simulink model "sdruFMReceiverSimulinkExample"  (R2019a)
settings: Solver=FixedStepDiscrete  StartTime=0.0  StopTime=inf  RelTol=1e-3
PreLoadFcn:
  | platform = sdruExampleFindRadio;
  | stereoFMRxParams = getParamsSdruFMExamples(platform);
  | clear platform
PostLoadFcn:
  | sdruExampleSetAvailableRadio();
InitFcn:
  | platform = get_param([gcs '/SDRu Receiver'], 'Platform');
  | stereoFMRxParams = getParamsSdruFMExamples(platform);
  | clear platform
libraries: simulink x1, dspsnks4 x1, commanabbnd3 x1, sdrublksprivate x1, commsdrhw_v2 x1
Description:
  | This model uses Universal Software Radio Peripheral (USRP) hardware with Simulink(R) to perform FM demodulation and stereo decoding.
settings Model: Creator=The MathWorks, Inc.  LastModifiedBy=ASUS
settings DataIOCC: SaveFormat=Structure  SaveOutput=off  SignalLogging=off  DSMLogging=off  SaveTime=off  ReturnWorkspaceOutputs=off
settings OptimizationCC: ExpressionDepthLimit=2147483647  EfficientMapNaN2IntZero=off  LifeSpan=inf  SimCompilerOptimization=on
settings DebuggingCC: UnderspecifiedInitializationDetection=Classic  MergeDetectMultiDrivingBlocksExec=none  SolverPrmCheckMsg=warning  InheritedTsInSrcMsg=none  MultiTaskCondExecSysMsg=none  ParameterPrecisionLossMsg=none  FcnCallInpInsideContextMsg=warning  AllowSymbolicDim=off  StateNameClashWarn=warning  SFUnexpectedBacktrackingDiag=warning  SFNoUnconditionalDefaultTransitionDiag=warning  SFExecutionAtInitializationDiag=none  ArithmeticOperatorsInVariantConditions=warning
settings HardwareCC: ProdBitPerPointer=32  ProdBitPerSizeT=32  ProdBitPerPtrDiffT=32  ProdLargestAtomicFloat=None  ProdIntDivRoundTo=Undefined  ProdEndianess=Unspecified  ProdWordSize=32  ProdHWDeviceType=32-bit Generic  TargetBitPerPointer=64  TargetBitPerSizeT=64  TargetBitPerPtrDiffT=64  TargetLongLongMode=on  TargetIntDivRoundTo=Zero  TargetEndianess=LittleEndian  TargetWordSize=64  TargetHWDeviceType=Generic->MATLAB Host Computer  ProdEqTarget=off
settings ModelReferenceCC: PropagateSignalLabelsOutOfModel=off
settings SFSimCC: SimIntegrity=off  SimUseLocalCustomCode=off
settings RTWCC: RTWUseLocalCustomCode=off
settings RTWCC: CustomSourceCode=|
  | #include <stdio.h>
  | #include <stdlib.h>
settings CodeAppCC: MaxIdLength=128  StateflowObjectComments=on
settings GRTTargetCC: TargetLangStandard=C89/C90 (ANSI)  GeneratePreprocessorConditionals=Disable all  CombineOutputUpdateFcns=off  GRTInterface=on
settings ConfigComp: CovMetricSettings=dw  CovHtmlReporting=on  CovSaveCumulativeToWorkspaceVar=on  CovSaveSingleToWorkspaceVar=on  CovExternalEMLEnable=off  CovSFcnEnable=off

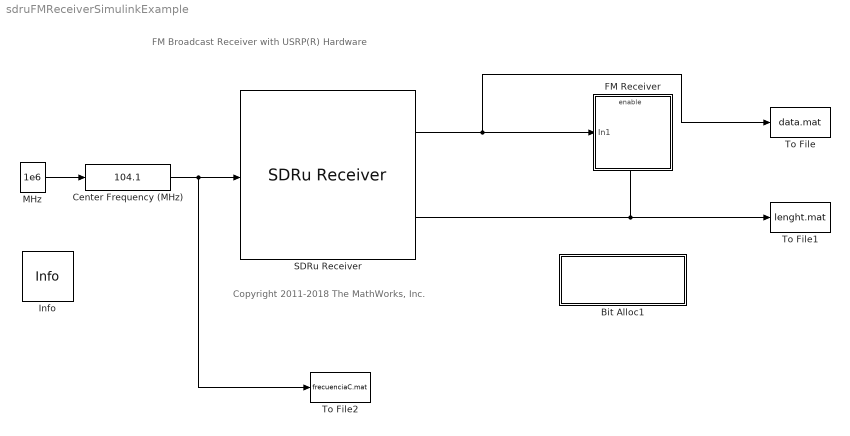
== system sdruFMReceiverSimulinkExample ==
  note: Copyright 2011-2018 The MathWorks, Inc.
  note: FM Broadcast Receiver with USRP(R) Hardware
  Bit Alloc1 : Subsystem
      settings: OpenFcn=sdruFMReceiverMidiSimulinkExample
      mask Display: disp('Alternative version\nwith midi controller\nfor station selection')
  Center Frequency (MHz) : simulink/Math Operations/Slider Gain  gain=104.1  low=87.5  high=108
  FM Receiver : Subsystem  TreatAsAtomicUnit=on
      mask Display:
      | plot(0,0,100,100,[5+4.5*[0:.15:10] 50 50 50 50+4.5*[0:10]],[85+10*[sin([0:.15:10]*pi*2+cumsum(sin([0:.15:10]*pi/5))/2)] 85 99 75   10*sin([0:10]*pi/5)+85])
      | disp('\nFM\nBroadcast\nDemodulator')
  Info : sdrublksprivate/Info  SystemSampleTime=-1
      settings: SourceProductName=Communications Toolbox Support Package for USRP Radio  SourceProductBaseCode=USRP
  MHz : Constant  Value=1e6  VectorParams1D=off  SampleTime=-1  FramePeriod=-1
  SDRu Receiver : commsdrhw_v2/SDRu Receiver  rxtx=rx  initializeIPAddress=0  devMap=0  USRP2_IP=192.168.10.2  USRP_IP_X300=192.168.10.2  USRP_IP_X310=192.168.10.2  USRP_serialNumB200=No devices found  USRP_serialNumB210=30ECBB4  platform=B210  prevPlatform=B210  lastIPAddressPopup=192.168.10.2  USRP_ID=30ECBB4  LastIPAddress=192.168.10.2  ChannelMapping=1  centerFrequencySrc=Input port  centerFrequency=2.45e9  loOffsetSrc=Dialog  loOffset=0  gainSrc=Dialog  gain=stereoFMRxParams.RadioGain  PPSSource=Internal  clockSource=Internal  masterClkRateParam=20000000  masterClkRateB200=stereoFMRxParams.RadioMasterClockRate  masterClkRateB210=stereoFMRxParams.RadioMasterClockRate  masterClkRateX300=200e6  masterClkRateX310=200e6  masterClkRate=100e6  decimInterpSrc=Dialog  decimInterp=stereoFMRxParams.RadioDecimationFactor  USRP2_IP_NUM=[51 48 69 67 66 66 52]  TransportDataType=int16  overrunUnderrunPort=off  sampleTime=1/stereoFMRxParams.RadioSampleRate  outputDatatype=single  frameLength=stereoFMRxParams.RadioFrameLength  HOST_DATA_PORT=30000  HOST_CONTROL_PORT=30002  USRP2_DATA_PORT=32769  USRP2_CONTROL_PORT=32768  bufferMode=Continuous streaming  EnableBurstMode=off  NumFramesInBurst=100
      settings: SourceProductName=Communications Toolbox Support Package for USRP Radio  SourceProductBaseCode=USRP
  To File : ToFile  Filename=data.mat  SaveFormat=Timeseries
  To File1 : ToFile  Filename=lenght.mat  SaveFormat=Timeseries
  To File2 : ToFile  Filename=frecuenciaC.mat  SaveFormat=Timeseries
  wires:
  SDRu Receiver/2 -> To File1/1, FM Receiver/Enable
  MHz/1 -> Center Frequency (MHz)/1
  SDRu Receiver/1 -> To File/1, FM Receiver/1(In1)
  Center Frequency (MHz)/1 -> To File2/1, SDRu Receiver/1

== system sdruFMReceiverSimulinkExample/Bit Alloc1 ==

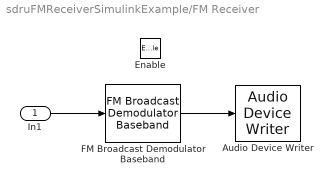
== system sdruFMReceiverSimulinkExample/FM Receiver ==
  In1 : Inport
  Enable : EnablePort
  Audio Device Writer : dspsnks4/Audio Device Writer  Driver=DirectSound  Device=Default  InheritSampleRate=on  SampleRate=44100  BitDepth=16-bit integer  BufferSize=4096  NumBuffers=10  DefaultOutputChannelMapping=on  OutputChannelMapping=1:2  OutputNumUnderrunSamples=off  DriverIdx=1  DeviceWarnFlag=''
  FM Broadcast Demodulator Baseband : commanabbnd3/FM Broadcast Demodulator Baseband  SampleRate=stereoFMRxParams.RadioSampleRate  FrequencyDeviation=stereoFMRxParams.FrequencyDeviation  FilterTimeConstant=stereoFMRxParams.FilterTimeConstant  AudioSampleRate=stereoFMRxParams.AudioSampleRate  PlaySound=off  BufferSize=stereoFMRxParams.BufferSize  Stereo=on  RBDS=off  RBDSSamplesPerSymbol=10  RBDSCostasLoop=off  SimulateUsing=Code generation
      settings: SourceProductName=Communications Toolbox  SourceProductBaseCode=CM
  wires:
  In1/1 -> FM Broadcast Demodulator Baseband/1
  FM Broadcast Demodulator Baseband/1 -> Audio Device Writer/1
